simulink model "AltitudeController"  (Simulink 8.5)
settings: Solver=ode45  StartTime=0.0  StopTime=20  RelTol=1e-3
libraries: simulink x7
settings Model: Creator=Suriya  LastModifiedBy=spachaimuthu
settings DebuggingCC: SolverPrmCheckMsg=warning  FcnCallInpInsideContextMsg=EnableAllAsWarning
settings GRTTargetCC: CombineOutputUpdateFcns=on  GRTInterface=off

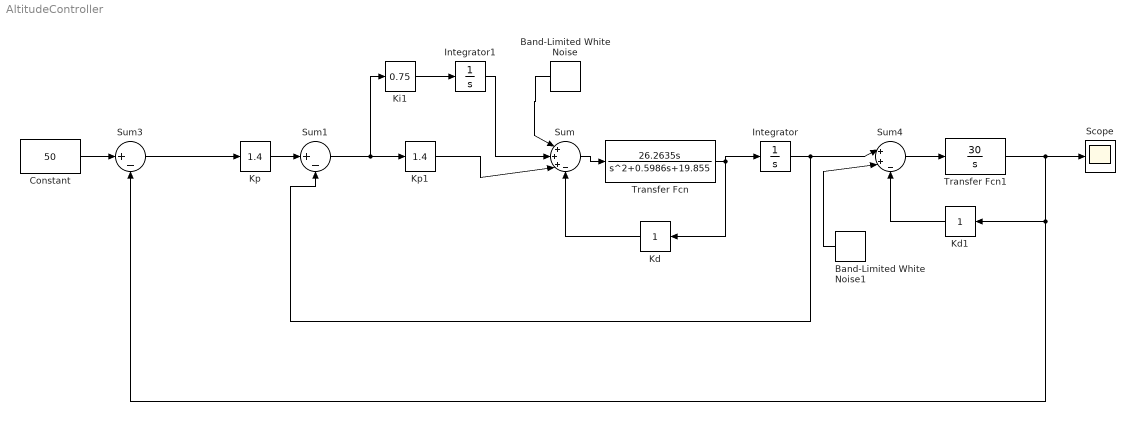
== system AltitudeController ==
  Band-Limited White Noise : simulink/Sources/Band-Limited White Noise  Cov=[0.1]  Ts=0.1  seed=[23341]
  Band-Limited White Noise1 : simulink/Sources/Band-Limited White Noise  Cov=[0.1]  Ts=0.1  seed=[23341]
  Constant : Constant  Value=50
  Integrator : Integrator
  Integrator1 : Integrator
  Kd : simulink/Math Operations/Slider Gain  low=0  gain=1  high=10
  Kd1 : simulink/Math Operations/Slider Gain  low=0  gain=1  high=10
  Ki1 : simulink/Math Operations/Slider Gain  low=0  gain=0.75  high=200
  Kp : simulink/Math Operations/Slider Gain  low=0  gain=1.4  high=150
  Kp1 : simulink/Math Operations/Slider Gain  low=0  gain=1.4  high=500
  Scope : Scope
  Sum : Sum  Inputs=|+++-
  Sum1 : Sum  Inputs=|+-
  Sum3 : Sum  Inputs=|+-
  Sum4 : Sum  Inputs=|++-
  Transfer Fcn : TransferFcn  Numerator=[26.2635 0]  Denominator=[1 0.5986 19.855]
  Transfer Fcn1 : TransferFcn  Numerator=[30]  Denominator=[1 0]
  wires:
  Sum/1 -> Transfer Fcn/1
  Ki1/1 -> Integrator1/1
  Transfer Fcn/1 -> Integrator/1, Kd/1
  Band-Limited White Noise/1 -> Sum/1
  Integrator1/1 -> Sum/2
  Kp1/1 -> Sum/3
  Kd/1 -> Sum/4
  Sum1/1 -> Kp1/1, Ki1/1
  Integrator/1 -> Sum1/2, Sum4/1
  Sum3/1 -> Kp/1
  Band-Limited White Noise1/1 -> Sum4/2
  Sum4/1 -> Transfer Fcn1/1
  Transfer Fcn1/1 -> Scope/1, Sum3/2, Kd1/1
  Constant/1 -> Sum3/1
  Kp/1 -> Sum1/1
  Kd1/1 -> Sum4/3
